simulink subsystem "Gsc"  (R2021b)
settings: Solver=VariableStepAuto  StartTime=0.0  StopTime=10.0  RelTol=1e-3
values from neighbouring files (symbols this model uses):
  kbb = 5*g*rarm/(L*7)    (= 0.41838605682)    [Main.m]    (also in Main_plaque_sphere.m = 0.543652363636; Main_poutre_sphere.m)
settings Model: Creator=sama1402  LastModifiedBy=sama1402

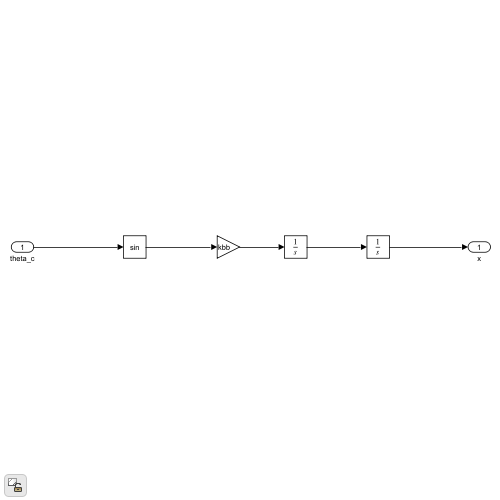
[thumbnail: Simulink's stored preview of the top-level diagram]
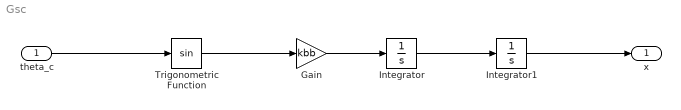
== system Gsc ==
  theta_c : Inport
  Gain : Gain  Gain=kbb
  Integrator : Integrator
  Integrator1 : Integrator
  Trigonometric Function : Trigonometry
  x : Outport
  wires:
  Trigonometric Function/1 -> Gain/1
  Gain/1 -> Integrator/1
  Integrator1/1 -> x/1
  Integrator/1 -> Integrator1/1
  theta_c/1 -> Trigonometric Function/1
